simulink model "Single_Phase_Diode_Rectifiers_100R"  (R2018a)
settings: Solver=FixedStepDiscrete  StartTime=0.0  StopTime=10.0  FixedStep=1.5e-3  MaxStep=0.2  RelTol=1e-4
libraries: powerlib x9
settings Model: Creator=Batuhan  LastModifiedBy=Batuhan
settings CodeAppCC: StateflowObjectComments=on

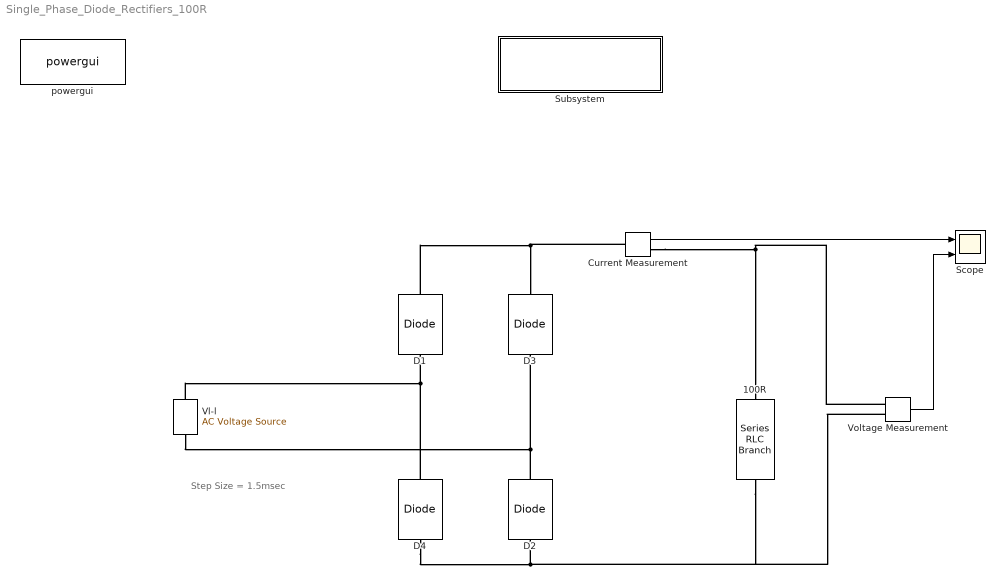
== system Single_Phase_Diode_Rectifiers_100R ==
  note: Step Size = 1.5msec
  100R : powerlib/Elements/Series RLC Branch  LConnTagsString=__new0  RConnTagsString=__new0  BranchType=R  Resistance=100  Inductance=1e-3  SetiL0=off  InitialCurrent=0  Capacitance=1e-6  Setx0=off  InitialVoltage=0  Measurements=None
  Current Measurement : powerlib/Measurements/Current Measurement  PhasorSimulation=off  OutputType=Complex  PSBequivalent=0
  D{1..4} (4 alike) : powerlib/Power Electronics/Diode  Ron=0.001  Lon=0  Vf=0.8  IC=0  UseSnubber=0  Rs=500  Cs=250e-9  Measurements=off
  Scope : Scope  NumInputPorts=2
  Subsystem : Subsystem
      settings: OpenFcn=open_system('power_new_palette')
      mask Display: disp(sprintf('Open Simscape Power Systems\n(Specialized Technology)\nPalette Library'));
  Vl-l : powerlib/Electrical Sources/AC Voltage Source  Amplitude=400  Phase=0  Frequency=50  SampleTime=0  Measurements=None  BusType=swing  Pref=10e3  Qref=0  Qmin=-inf  Qmax=+inf
  Voltage Measurement : powerlib/Measurements/Voltage Measurement  PhasorSimulation=off  OutputType=Complex  PSBequivalent=0
  powergui : powerlib/powergui  Priority=1  SimulationMode=Discrete  SampleTime=1.5e-3  frequency=60  Iterations=50  frequencyindice=50  Pbase=100e6  ErrMax=1e-4  UnitsV=kV  UnitsW=MW  buscounter=0  FunctionMessages=off  echomessages=off  EnableUseOfTLC=off  CurrentSourceSwitches=off  DisableSnubberDevices=off  DisableRonSwitches=off  DisableVfSwitches=off  DisplayEquations=off  SolverType=Tustin/Backward Euler (TBE)  Interpol=off  ExternalGateDelay=off  methode=off  Ts=100  x0status=blocks  SPID=on  SwTol=0  HookPort=off  RestoreLinks=warning  ResistiveCurrentMeasurement=off  Frange=[0:2:500]  Ylog=off  Xlog=on  ShowGrid=off  save=off  variable=ZData  structure=0  ZoomFFT=off  StartTime=0.0  cycles=1  DisplayStyle=1  fundamental=60  FreqAxis=off  MaxFrequency=1000  frequencyindicesteady=1  RmsSteady=1  display=off
  wires:
  Current Measurement/1 -> Scope/1
  Voltage Measurement/1 -> Scope/2
  connections:
  D2/RConn1 -- Vl-l/LConn1 -- D3/LConn1
  D4/RConn1 -- Vl-l/RConn1 -- D1/LConn1
  D1/RConn1 -- Current Measurement/LConn1 -- D3/RConn1
  D4/LConn1 -- 100R/RConn1 -- Voltage Measurement/LConn2 -- D2/LConn1
  Voltage Measurement/LConn1 -- Current Measurement/RConn1 -- 100R/LConn1

== system Single_Phase_Diode_Rectifiers_100R/Subsystem ==
